simulink model "GFLIB_Lut2D_BAM_F32"  (Simulink 8.3)
settings: Solver=ode45  StartTime=0.0  StopTime=10.0  RelTol=1e-3
undefined symbols (not defined in the file): pf32Table, s32MidIdx, u32ShamOffset1, u32ShamOffset2
settings Model: Creator=B17364  LastModifiedBy=B17364
settings OptimizationCC: ExpressionDepthLimit=2147483647
settings DebuggingCC: FcnCallInpInsideContextMsg=UseLocalSettings  StrictBusMsg=Warning

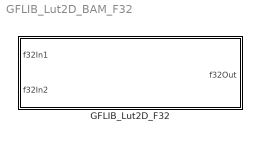
== system GFLIB_Lut2D_BAM_F32 ==
  GFLIB_Lut2D_F32 : Subsystem  mask(GFLIB_Lut2D_F32){u32ShamOffset1=u32ShamOffset1, u32ShamOffset2=u32ShamOffset2, pf32Table=pf32Table, s32MidIdx=s32MidIdx}
      mask help: Bit accurate model of Lut2D function.
      mask init:
      | pos = get_param(gcb, 'Position');width = pos(3) - pos(1); height = pos(4) - pos(2);tX=width/2;tY=height*0.9;
      mask Display: color('black');port_label('input',1,'f32In1');port_label('input',2,'f32In2');port_label('output',1,'f32Out');color('black');disp('GFLIB_Lut2D_F32');color('blue');text(tX,tY, 'BAM', 'horizontalAlignment', 'center');

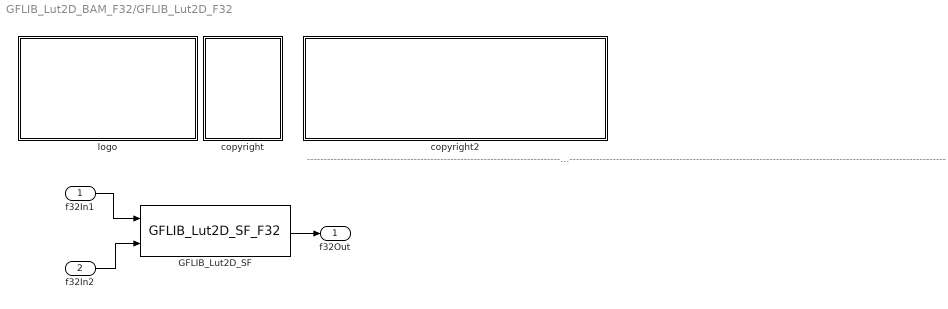
== system GFLIB_Lut2D_BAM_F32/GFLIB_Lut2D_F32 ==
  note: ---------------------------------------------------------------------------------------------------------------------------------------------------------------------------------------------------
  f32In1 : Inport
  f32In2 : Inport  Port=2
  GFLIB_Lut2D_SF : S-Function  FunctionName=GFLIB_Lut2D_SF_F32  Parameters=u32ShamOffset1,u32ShamOffset2,pf32Table,s32MidIdx  EnableBusSupport=off
  copyright : Subsystem
      mask Display:
      | text(10,90,'FILE:');text(10,75,'DESRIPTION:')
      | text(10,60,'COPYRIGHT:')
      | text(10,45,'VERSION:')
      | text(10,30,'DATE:')
  copyright2 : Subsystem
      mask Display:
      | text(10,90,'GFLIB_Lut2D_BAM_F32.mdl');text(10,75,'Two dimensional Look-up table function');text(10,60,'Freescale')
      | text(10,45,'0.1');text(10,30,'17-Jun-2013');
  logo : Subsystem
      mask Display: image(imread('logo.jpg'))
  f32Out : Outport
  wires:
  f32In1/1 -> GFLIB_Lut2D_SF/1
  f32In2/1 -> GFLIB_Lut2D_SF/2
  GFLIB_Lut2D_SF/1 -> f32Out/1

== system GFLIB_Lut2D_BAM_F32/GFLIB_Lut2D_F32/copyright ==

== system GFLIB_Lut2D_BAM_F32/GFLIB_Lut2D_F32/copyright2 ==

== system GFLIB_Lut2D_BAM_F32/GFLIB_Lut2D_F32/logo ==
